simulink model "cartesianControl6Ranalytical"  (R2023b)
settings: Solver=FixedStepAuto  StartTime=0.0  StopTime=5  FixedStep=0.001  RelTol=1e-3
values from neighbouring files (symbols this model uses):
  Kp = eye(sizeTaskSpace,sizeTaskSpace)    [cartesianControl6Rmain.m]
  myRob = loadrobot("abbIrb120")    [cartesianControl6Rmain.m]
  orie_f = tform2rotm(makehgtform('yrotate',pi/2))    [cartesianControl6Rmain.m]
  orie_i = tform2rotm(initialPose)    [cartesianControl6Rmain.m]
  pe_f = [pe_f; zHeight_ideal]    [cartesianControl6Rmain.m]
  pe_i = transpose(tform2trvec(initialPose))    [cartesianControl6Rmain.m]
  q0 = configSol    [cartesianControl6Rmain.m]
  t_f = 5    [cartesianControl6Rmain.m]
  t_i = 0    [cartesianControl6Rmain.m]
undefined symbols (not defined in the file or in its folder): DiscIntNeverNeededParam
settings Model: Creator=ggi01  LastModifiedBy=ggi01
settings SolverCC: AlgebraicLoopSolver=TrustRegion
settings DebuggingCC: UnconnectedInputMsg=warning  UnconnectedOutputMsg=warning  UnconnectedLineMsg=warning
settings ModelReferenceCC: EnableRefExpFcnMdlSchedulingChecks=on
settings RTWCC: DLArmComputeVersion=19.05

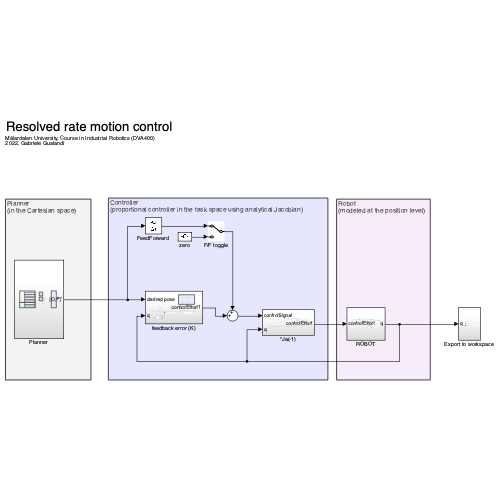
[thumbnail: Simulink's stored preview of the top-level diagram]
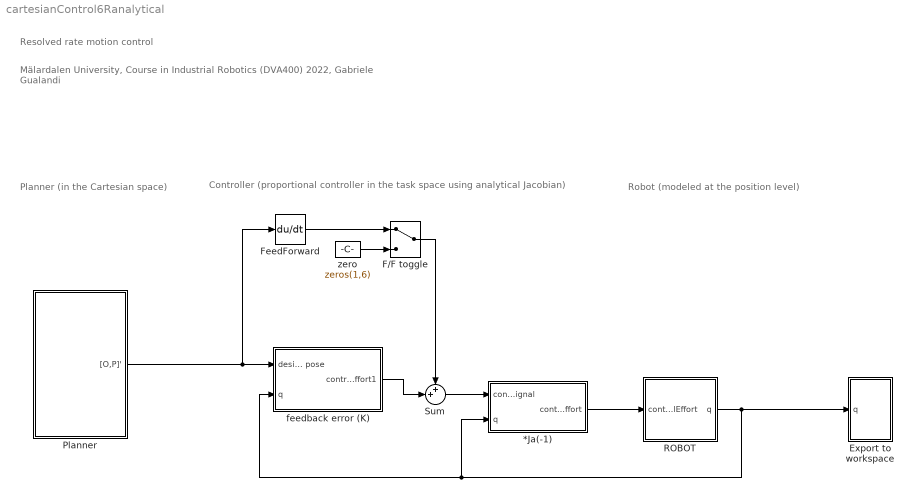
== system cartesianControl6Ranalytical ==
  note: Mälardalen University, Course in Industrial Robotics (DVA400)
      | 2022, Gabriele Gualandi
  note: Resolved rate motion control
  note: Robot
      | (modeled at the position level)
  note: Planner
      | (in the Cartesian space)
  note: Controller
      | (proportional controller in the task space using analytical Jacobian)
  *Ja(-1) : Subsystem
  Export to workspace : Subsystem
  F/F toggle : ManualSwitch
  FeedForward : Derivative
  Planner : Subsystem
  ROBOT : Subsystem
  Sum : Sum  Inputs=++|
  feedback error (K) : Subsystem
  zero : Constant  Value=zeros(1,6)
  wires:
  FeedForward/1 -> F/F toggle/1
  feedback error (K)/1(controlEffort1) -> Sum/2
  Sum/1 -> *Ja(-1)/1(controlSignal)
  *Ja(-1)/1(controlEffort) -> ROBOT/1(controlEffort)
  F/F toggle/1 -> Sum/1
  zero/1 -> F/F toggle/2
  ROBOT/1(q) -> Export to workspace/1(q), *Ja(-1)/2(q), feedback error (K)/2(q)
  Planner/1("[O,P]'") -> FeedForward/1, feedback error (K)/1(desired pose)

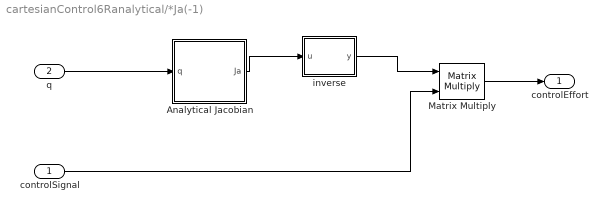
== system cartesianControl6Ranalytical/*Ja(-1) ==
  controlSignal : Inport
  q : Inport  Port=2
  Analytical Jacobian : Subsystem
  Matrix Multiply : Product  Multiplication=Matrix(*)
  inverse : MATLAB Function  TreatAsAtomicUnit=on
  controlEffort : Outport
  wires:
  q/1 -> Analytical Jacobian/1(q)
  controlSignal/1 -> Matrix Multiply/2
  inverse/1(y) -> Matrix Multiply/1
  Analytical Jacobian/1(Ja) -> inverse/1(u)
  Matrix Multiply/1 -> controlEffort/1

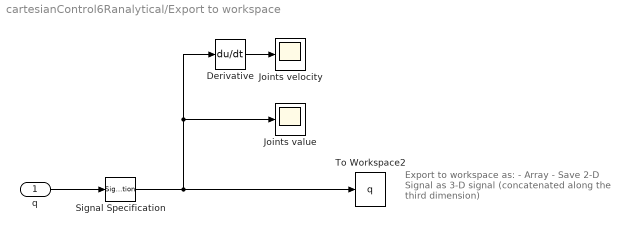
== system cartesianControl6Ranalytical/Export to workspace ==
  note: Export to workspace as:
      | - Array
      | - Save 2-D Signal as 3-D signal
      | (concatenated along the third dimension)
  q : Inport
  Derivative : Derivative
  Joints value : Scope
  Joints velocity : Scope
  Signal Specification : SignalSpecification  Dimensions=[6,1]
  To Workspace2 : ToWorkspace  VariableName=q  SampleTime=-1
  wires:
  Derivative/1 -> Joints velocity/1
  q/1 -> Signal Specification/1
  Signal Specification/1 -> Joints value/1, Derivative/1, To Workspace2/1

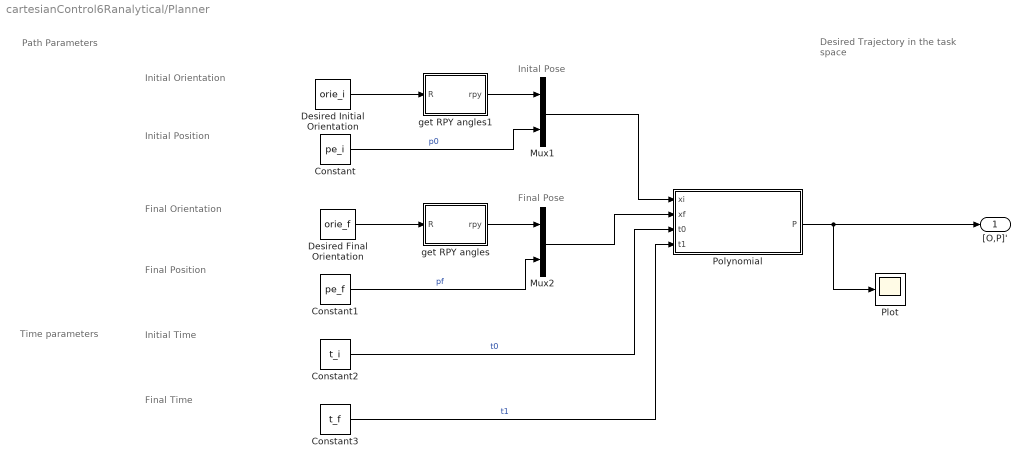
== system cartesianControl6Ranalytical/Planner ==
  note: Desired Trajectory
      | in the task space
  note: Time parameters
  note: Path Parameters
  note: Inital Pose
  note: Initial Orientation
  note: Initial Position
  note: Final Orientation
  note: Final Position
  note: Initial Time
  note: Final Time
  note: Final Pose
  Constant : Constant  Value=pe_i  VectorParams1D=off
  Constant1 : Constant  Value=pe_f  VectorParams1D=off
  Constant2 : Constant  Value=t_i
  Constant3 : Constant  Value=t_f
  Desired Final Orientation : Constant  Value=orie_f
  Desired Initial Orientation : Constant  Value=orie_i
  Mux1 : Mux  Inputs=2
  Mux2 : Mux  Inputs=2
  Plot : Scope
  Polynomial : Subsystem
  get RPY angles : MATLAB Function  TreatAsAtomicUnit=on
  get RPY angles1 : MATLAB Function  TreatAsAtomicUnit=on
  "[O,P]'" : Outport
  wires:
  Constant3/1 -> Polynomial/4(t1)  "t1"
  Constant2/1 -> Polynomial/3(t0)  "t0"
  Desired Final Orientation/1 -> get RPY angles/1(R)
  Polynomial/1(P) -> "[O,P]'"/1, Plot/1
  Desired Initial Orientation/1 -> get RPY angles1/1(R)
  Mux1/1 -> Polynomial/1(xi)
  Mux2/1 -> Polynomial/2(xf)
  get RPY angles1/1(rpy) -> Mux1/1
  Constant/1 -> Mux1/2  "p0"
  Constant1/1 -> Mux2/2  "pf"
  get RPY angles/1(rpy) -> Mux2/1

== system cartesianControl6Ranalytical/ROBOT ==
  controlEffort : Inport
  Constant : Constant  Value=q0
  Discrete-Time Integrator : DiscreteIntegrator  InitialConditionSource=external  SampleTime=-1  ICPrevOutput=DiscIntNeverNeededParam  ICPrevScaledInput=DiscIntNeverNeededParam
  Saturation : Saturate  UpperLimit=inf  LowerLimit=-inf
  q : Outport
  wires:
  Discrete-Time Integrator/1 -> q/1  "q"
  controlEffort/1 -> Saturation/1
  Constant/1 -> Discrete-Time Integrator/2
  Saturation/1 -> Discrete-Time Integrator/1

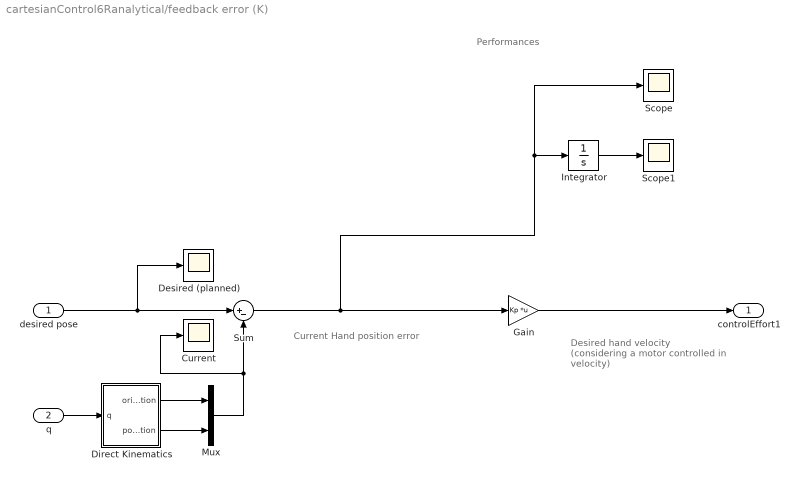
== system cartesianControl6Ranalytical/feedback error (K) ==
  note: Performances
  note: Current Hand position error
  note: Desired hand velocity
      | (considering a motor controlled
      | in velocity)
  desired pose : Inport
  q : Inport  Port=2
  Current : Scope
  Desired (planned) : Scope
  Direct Kinematics : Subsystem
  Gain : Gain  Gain=Kp  Multiplication=Matrix(K*u)
  Integrator : Integrator
  Mux : Mux  Inputs=2
  Scope : Scope
  Scope1 : Scope
  Sum : Sum  Inputs=|+-
  controlEffort1 : Outport
  wires:
  q/1 -> Direct Kinematics/1(q)
  Direct Kinematics/1(orientation) -> Mux/1
  Direct Kinematics/2(position) -> Mux/2
  desired pose/1 -> Desired (planned)/1, Sum/1
  Mux/1 -> Sum/2, Current/1
  Gain/1 -> controlEffort1/1
  Sum/1 -> Scope/1, Integrator/1, Gain/1
  Integrator/1 -> Scope1/1

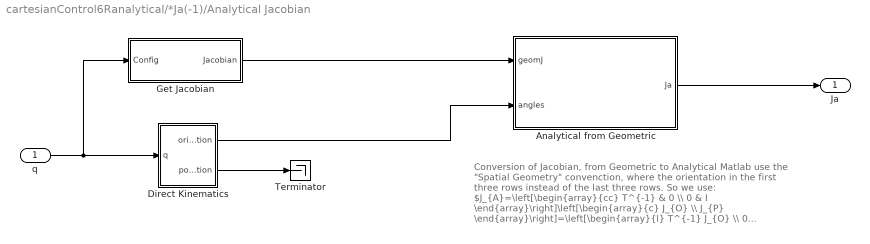
== system cartesianControl6Ranalytical/*Ja(-1)/Analytical Jacobian ==
  note: Conversion of Jacobian, from Geometric to Analytical
      |
      | Matlab use the "Spatial Geometry" convenction, where the orientation in the first three rows instead of the last three rows. So we use:
      |
      | $J_{A}=\left[\begin{array}{cc} T^{-1} & 0 \\ 0 & I \end{array}\right]\left[\begin{array}{c} J_{O} \\ J_{P} \end{array}\right]=\left[\begin{array}{l} T^{-1} J_{O} \\ 0 \end{array}\right]+\left[\begin{array}{c} 0\\ J_{P} \end{array}\right] \quad \text {if } \,\, J=\left[\begin{array}{l} J_{O} \\ J_{P} \end{array}\right]$
      |
      | If orientation is in the last three rows (as in most of the text books) we would use instead:
      |
      | $J_{A}=\left[\begin{array}{cc} I & 0 \\ 0 & T^{-1} \end{array}\right]\left[\begin{array}{c} J_{P} \\ J_{O} \end{array}\right]=\left[\begin{array}{l} J_{P} \\ 0 \end{array}\right]+\left[\begin{array}{c} 0\\ T^{-1} J_{O} \end{array}\right] \quad \text { if } \,\, J=\left[\begin{array}{l} J_{P} \\ J_{O} \end{array}\right]$
  q : Inport
  Analytical from Geometric : MATLAB Function  TreatAsAtomicUnit=on
  Direct Kinematics : Subsystem
  Get Jacobian : Subsystem  mask(Get Jacobian){RigidBodyTree=myRob, EndEffector=tool0, SimulateUsing=Code generation}
      mask prompts: RigidBodyTree "robotics:robotslmanip:blockmask:RigidBodyTreePrompt"; EndEffector "robotics:robotslmanip:blockmask:EndEffectorPrompt"; SimulateUsing "SystemBlock:MATLABSystem:SimulateUsing"
      mask help: robotics:robotslmanip:blockmask:GetJacobianDescription
      mask init:
      | try
      |    [TreeStruct, NumBodies, sysName] = robotics.slmanip.internal.block.RBTAlgorithmBlockMasks.updateMaskWorkSpaceVariables(gcb, RigidBodyTree);
      |    robotics.slmanip.internal.block.RBTAlgorithmBlockMasks.updateBlockInputDimensions(gcb, TreeStruct, 'Config');
      | catch ME
      |    TreeStruct = [];  NumBodies = [];   sysName = '???';
      |    throw(ME);
      | end
      | EndEffectorArray = robotics.slmanip.internal.block.RBTAlgorithmBlockMasks.updateBodyWSVar(gcb, RigidBodyTree, 'EndEffector');
      settings: LibrarySourceBlock=robotmaniplib/Get Jacobian
      mask Help: helpview(fullfile(docroot,'robotics','helptargets.map'), 'rstGetJacobian');
      mask TypeOptions SimulateUsing: MATLAB System/SimulateUsing
      mask DialogControl RigidBodyTree Prompt: Rigid body tree:
      mask DialogControl EndEffector Prompt: End effector:
      mask DialogControl ListControl Prompt: robotics:robotslmanip:blockmask:SelectBodyButtonPrompt
      mask DialogControl ListControl Callback: robotics.slmanip.internal.block.RBTAlgorithmBlockMasks.updateMaskBodyList(gcb, 'EndEffector');
      mask DialogControl SimulateUsing Prompt: Simulate using:
      mask DialogControl SimulateUsing Tooltip: SystemBlock:MATLABSystem:SimulateUsingDescription
      mask Display:
      | if (strcmp(sysName,'???'))
      | 	color('red');
      | else
      |     color('blue');
      | end
      | text(0.99, 0.99, sysName, 'horizontalAlignment', 'right', 'verticalAlignment','top');
      | 
      | color('black');
      | DescText = ['EE: ' get_param(gcb,'EndEffector')];
      | text(0.5, 0.05, DescText, 'horizontalAlignment', 'center', 'verticalAlignment','bottom');
      | 
      | port_label('input', 1, 'Config')
      | port_label('output', 1, 'Jacobian')
  Terminator : Terminator
  Ja : Outport
  wires:
  Direct Kinematics/1(orientation) -> Analytical from Geometric/2(angles)
  Direct Kinematics/2(position) -> Terminator/1
  Analytical from Geometric/1(Ja) -> Ja/1
  Get Jacobian/1(Jacobian) -> Analytical from Geometric/1(geomJ)
  q/1 -> Get Jacobian/1(Config), Direct Kinematics/1(q)

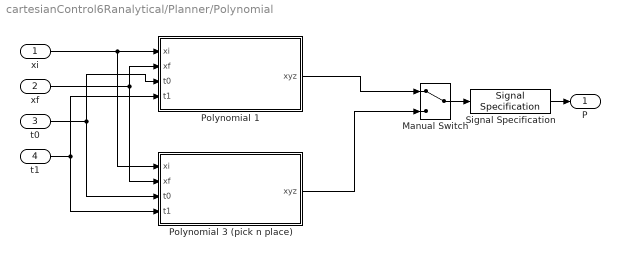
== system cartesianControl6Ranalytical/Planner/Polynomial ==
  xi : Inport
  xf : Inport  Port=2
  t0 : Inport  Port=3
  t1 : Inport  Port=4
  Manual Switch : ManualSwitch
  Polynomial 1 : Subsystem
  Polynomial 3 (pick n place) : Subsystem
  Signal Specification : SignalSpecification  OutDataTypeStr=double  Dimensions=[6,1]
  P : Outport
  wires:
  Polynomial 1/1(xyz) -> Manual Switch/1
  Polynomial 3 (pick n place)/1(xyz) -> Manual Switch/2
  xi/1 -> Polynomial 3 (pick n place)/1(xi), Polynomial 1/1(xi)
  xf/1 -> Polynomial 3 (pick n place)/2(xf), Polynomial 1/2(xf)
  t0/1 -> Polynomial 1/3(t0), Polynomial 3 (pick n place)/3(t0)
  t1/1 -> Polynomial 3 (pick n place)/4(t1), Polynomial 1/4(t1)
  Manual Switch/1 -> Signal Specification/1
  Signal Specification/1 -> P/1

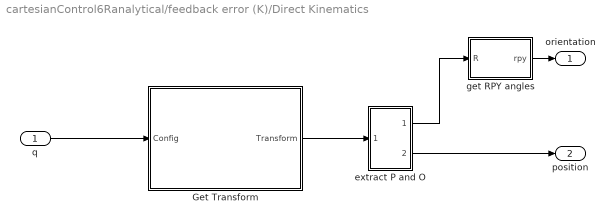
== system cartesianControl6Ranalytical/feedback error (K)/Direct Kinematics ==
  q : Inport
  Get Transform : Subsystem  mask(Get Transform){RigidBodyTree=myRob, SourceBody=tool0, TargetBody=base, SimulateUsing=Code generation}
      mask prompts: RigidBodyTree "robotics:robotslmanip:blockmask:RigidBodyTreePrompt"; SourceBody "robotics:robotslmanip:blockmask:GetTransformSourceBodyPrompt"; TargetBody "robotics:robotslmanip:blockmask:GetTransformTargetBodyPrompt"; SimulateUsing "SystemBlock:MATLABSystem:SimulateUsing"
      mask help: robotics:robotslmanip:blockmask:GetTransformDescription
      mask init:
      | try
      |    [TreeStruct, NumBodies, sysName] = robotics.slmanip.internal.block.RBTAlgorithmBlockMasks.updateMaskWorkSpaceVariables(gcb, RigidBodyTree);
      |    robotics.slmanip.internal.block.RBTAlgorithmBlockMasks.updateBlockInputDimensions(gcb, TreeStruct, 'Config');
      | catch ME
      |    TreeStruct = [];  NumBodies = [];   sysName = '???';
      |    throw(ME);
      | end
      | SourceBodyArray = robotics.slmanip.internal.block.RBTAlgorithmBlockMasks.updateBodyWSVar(gcb, RigidBodyTree, 'SourceBody');
      | TargetBodyArray = robotics.slmanip.internal.block.RBTAlgorithmBlockMasks.updateBodyWSVar(gcb, RigidBodyTree, 'TargetBody');
      settings: LibrarySourceBlock=robotmaniplib/Get Transform
      mask Help: helpview(fullfile(docroot,'robotics','helptargets.map'), 'rstGetTransform');
      mask TypeOptions SimulateUsing: MATLAB System/SimulateUsing
      mask DialogControl RigidBodyTree Prompt: Rigid body tree:
      mask DialogControl SourceBody Prompt: Source body:
      mask DialogControl ListControl1 Prompt: Select body >>
      mask DialogControl ListControl1 Callback: robotics.slmanip.internal.block.RBTAlgorithmBlockMasks.updateMaskBodyList(gcb, 'SourceBody');
      mask DialogControl TargetBody Prompt: Target body:
      mask DialogControl ListControl2 Prompt: Select body >>
      mask DialogControl ListControl2 Callback: robotics.slmanip.internal.block.RBTAlgorithmBlockMasks.updateMaskBodyList(gcb, 'TargetBody');
      mask DialogControl SimulateUsing Prompt: Simulate using:
      mask DialogControl SimulateUsing Tooltip: SystemBlock:MATLABSystem:SimulateUsingDescription
      mask Display:
      | if (strcmp(sysName,'???'))
      | 	color('red');
      | else
      |     color('blue');
      | end
      | text(0.99, 0.99, sysName, 'horizontalAlignment', 'right', 'verticalAlignment','top');
      | 
      | color('black')
      | SourceText = ['Source: ' get_param(gcb,'SourceBody')];
      | TargetText = ['Target: ' get_param(gcb,'TargetBody')];
      | DescText = [SourceText newline TargetText];
      | text(0.5, 0.05, DescText, 'horizontalAlignment', 'center','verticalAlignment','bottom');
      | 
      | port_label('input', 1, 'Config')
      | port_label('output', 1, 'Transform')
  extract P and O : Subsystem
  get RPY angles : MATLAB Function  TreatAsAtomicUnit=on
  orientation : Outport
  position : Outport  Port=2
  wires:
  get RPY angles/1(rpy) -> orientation/1
  extract P and O/1(orientation) -> get RPY angles/1(R)
  extract P and O/2(position) -> position/1
  Get Transform/1(Transform) -> extract P and O/1(In1)
  q/1 -> Get Transform/1(Config)

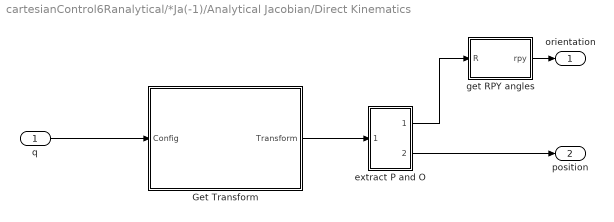
== system cartesianControl6Ranalytical/*Ja(-1)/Analytical Jacobian/Direct Kinematics ==
  q : Inport
  Get Transform : Subsystem  mask(Get Transform){RigidBodyTree=myRob, SourceBody=tool0, TargetBody=base, SimulateUsing=Code generation}
      mask prompts: RigidBodyTree "robotics:robotslmanip:blockmask:RigidBodyTreePrompt"; SourceBody "robotics:robotslmanip:blockmask:GetTransformSourceBodyPrompt"; TargetBody "robotics:robotslmanip:blockmask:GetTransformTargetBodyPrompt"; SimulateUsing "SystemBlock:MATLABSystem:SimulateUsing"
      mask help: robotics:robotslmanip:blockmask:GetTransformDescription
      mask init: same as cartesianControl6Ranalytical/feedback error (K)/Direct Kinematics/Get Transform
      settings: LibrarySourceBlock=robotmaniplib/Get Transform
      mask Help: helpview(fullfile(docroot,'robotics','helptargets.map'), 'rstGetTransform');
      mask TypeOptions SimulateUsing: MATLAB System/SimulateUsing
      mask DialogControl RigidBodyTree Prompt: Rigid body tree:
      mask DialogControl SourceBody Prompt: Source body:
      mask DialogControl ListControl1 Prompt: Select body >>
      mask DialogControl ListControl1 Callback: robotics.slmanip.internal.block.RBTAlgorithmBlockMasks.updateMaskBodyList(gcb, 'SourceBody');
      mask DialogControl TargetBody Prompt: Target body:
      mask DialogControl ListControl2 Prompt: Select body >>
      mask DialogControl ListControl2 Callback: robotics.slmanip.internal.block.RBTAlgorithmBlockMasks.updateMaskBodyList(gcb, 'TargetBody');
      mask DialogControl SimulateUsing Prompt: Simulate using:
      mask DialogControl SimulateUsing Tooltip: SystemBlock:MATLABSystem:SimulateUsingDescription
      mask Display:
      | if (strcmp(sysName,'???'))
      | 	color('red');
      | else
      |     color('blue');
      | end
      | text(0.99, 0.99, sysName, 'horizontalAlignment', 'right', 'verticalAlignment','top');
      | 
      | color('black')
      | SourceText = ['Source: ' get_param(gcb,'SourceBody')];
      | TargetText = ['Target: ' get_param(gcb,'TargetBody')];
      | DescText = [SourceText newline TargetText];
      | text(0.5, 0.05, DescText, 'horizontalAlignment', 'center','verticalAlignment','bottom');
      | 
      | port_label('input', 1, 'Config')
      | port_label('output', 1, 'Transform')
  extract P and O : Subsystem
  get RPY angles : MATLAB Function  TreatAsAtomicUnit=on
  orientation : Outport
  position : Outport  Port=2
  wires:
  get RPY angles/1(rpy) -> orientation/1
  extract P and O/1(orientation) -> get RPY angles/1(R)
  extract P and O/2(position) -> position/1
  Get Transform/1(Transform) -> extract P and O/1(In1)
  q/1 -> Get Transform/1(Config)

== system cartesianControl6Ranalytical/*Ja(-1)/Analytical Jacobian/Get Jacobian ==
  Config : Inport
  MATLAB System : MATLABSystem  System=robotics.slmanip.internal.block.GetJacobianBlock  TreeStruct=TreeStruct  EEBodyName=EndEffector  SimulateUsing=Code generation
      mask Type: robotics.slmanip.internal.block.GetJacobianBlock
      mask Display:
      | disp('GetJacobianBlock');
      | port_label('input',1,'q');
      | port_label('output',1,'jacobianMat');
  Jacobian : Outport  VectorParamsAs1DForOutWhenUnconnected=off
  wires:
  MATLAB System/1 -> Jacobian/1
  Config/1 -> MATLAB System/1

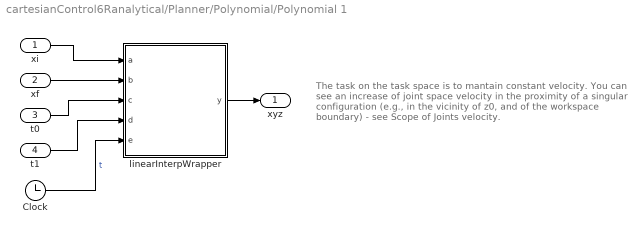
== system cartesianControl6Ranalytical/Planner/Polynomial/Polynomial 1 ==
  note: The task on the task space is to mantain constant velocity.
      | You can see an increase of joint space velocity in the proximity
      | of a singular configuration (e.g., in the vicinity of z0, and of the
      | workspace boundary) - see Scope of Joints velocity.
  xi : Inport
  xf : Inport  Port=2
  t0 : Inport  Port=3
  t1 : Inport  Port=4
  Clock : Clock
  linearInterpWrapper : MATLAB Function  TreatAsAtomicUnit=on
  xyz : Outport
  wires:
  t0/1 -> linearInterpWrapper/3(c)
  xi/1 -> linearInterpWrapper/1(a)
  xf/1 -> linearInterpWrapper/2(b)
  t1/1 -> linearInterpWrapper/4(d)
  Clock/1 -> linearInterpWrapper/5(e)  "t"
  linearInterpWrapper/1(y) -> xyz/1

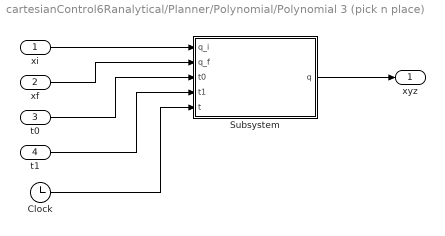
== system cartesianControl6Ranalytical/Planner/Polynomial/Polynomial 3 (pick n place) ==
  xi : Inport
  xf : Inport  Port=2
  t0 : Inport  Port=3
  t1 : Inport  Port=4
  Clock : Clock
  Subsystem : Subsystem
  xyz : Outport
  wires:
  Subsystem/1(q) -> xyz/1
  xf/1 -> Subsystem/2(q_f)
  Clock/1 -> Subsystem/5(t)
  t0/1 -> Subsystem/3(t0)
  xi/1 -> Subsystem/1(q_i)
  t1/1 -> Subsystem/4(t1)

== system cartesianControl6Ranalytical/feedback error (K)/Direct Kinematics/Get Transform ==
  Config : Inport
  MATLAB System : MATLABSystem  System=robotics.slmanip.internal.block.GetTransformBlock  TreeStruct=TreeStruct  SourceBodyName=SourceBody  TargetBodyName=TargetBody  SimulateUsing=Code generation
      mask Type: robotics.slmanip.internal.block.GetTransformBlock
      mask Display:
      | disp('GetTransformBlock');
      | port_label('input',1,'q');
      | port_label('output',1,'tform');
  Transform : Outport  VectorParamsAs1DForOutWhenUnconnected=off
  wires:
  MATLAB System/1 -> Transform/1
  Config/1 -> MATLAB System/1

== system cartesianControl6Ranalytical/feedback error (K)/Direct Kinematics/extract P and O ==
  In1 : Inport
  Orientation : MATLABFcn  MATLABFcn=tform2rotm  Output1D=off
  Position : MATLABFcn  MATLABFcn=tform2trvec
  orientation : Outport
  position : Outport  Port=2
  wires:
  Orientation/1 -> orientation/1
  In1/1 -> Position/1, Orientation/1
  Position/1 -> position/1

== system cartesianControl6Ranalytical/*Ja(-1)/Analytical Jacobian/Direct Kinematics/Get Transform ==
  Config : Inport
  MATLAB System : MATLABSystem  System=robotics.slmanip.internal.block.GetTransformBlock  TreeStruct=TreeStruct  SourceBodyName=SourceBody  TargetBodyName=TargetBody  SimulateUsing=Code generation
      mask Type: robotics.slmanip.internal.block.GetTransformBlock
      mask Display:
      | disp('GetTransformBlock');
      | port_label('input',1,'q');
      | port_label('output',1,'tform');
  Transform : Outport  VectorParamsAs1DForOutWhenUnconnected=off
  wires:
  MATLAB System/1 -> Transform/1
  Config/1 -> MATLAB System/1

== system cartesianControl6Ranalytical/*Ja(-1)/Analytical Jacobian/Direct Kinematics/extract P and O ==
  In1 : Inport
  Orientation : MATLABFcn  MATLABFcn=tform2rotm  Output1D=off
  Position : MATLABFcn  MATLABFcn=tform2trvec
  orientation : Outport
  position : Outport  Port=2
  wires:
  Orientation/1 -> orientation/1
  In1/1 -> Position/1, Orientation/1
  Position/1 -> position/1

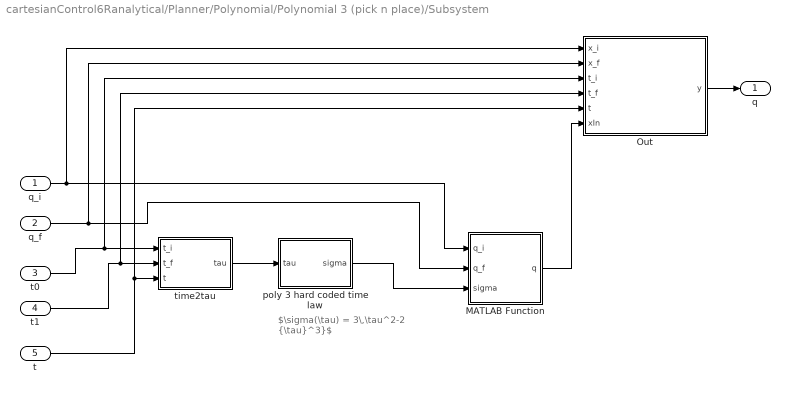
== system cartesianControl6Ranalytical/Planner/Polynomial/Polynomial 3 (pick n place)/Subsystem ==
  note: $\sigma(\tau) = 3\,\tau^2-2 {\tau}^3}$
  q_i : Inport
  q_f : Inport  Port=2
  t0 : Inport  Port=3
  t1 : Inport  Port=4
  t : Inport  Port=5
  MATLAB Function : MATLAB Function  TreatAsAtomicUnit=on
  Out : MATLAB Function  TreatAsAtomicUnit=on
  poly 3 hard coded time law : MATLAB Function  TreatAsAtomicUnit=on
  time2tau : MATLAB Function  TreatAsAtomicUnit=on
  q : Outport
  wires:
  q_f/1 -> Out/2(x_f), MATLAB Function/2(q_f)
  t/1 -> Out/5(t), time2tau/3(t)
  t0/1 -> Out/3(t_i), time2tau/1(t_i)
  MATLAB Function/1(q) -> Out/6(xIn)
  t1/1 -> Out/4(t_f), time2tau/2(t_f)
  q_i/1 -> Out/1(x_i), MATLAB Function/1(q_i)
  time2tau/1(tau) -> poly 3 hard coded time law/1(tau)
  poly 3 hard coded time law/1(sigma) -> MATLAB Function/3(sigma)
  Out/1(y) -> q/1

== matlab function cartesianControl6Ranalytical/Planner/Polynomial/Polynomial 3 (pick n place)/Subsystem/Out ==
  data: x_i input; y output; x_f input; t_i input; t_f input; t input; xIn input
function y = intervalGuardWrapper(x_i, x_f, t_i, t_f, t, xIn )

y = intervalGuard(x_i, x_f, t_i, t_f, t, xIn );

== matlab function cartesianControl6Ranalytical/*Ja(-1)/inverse ==
  data: u input; y output
function y = fcn(u)

y = inv(u);

== matlab function cartesianControl6Ranalytical/*Ja(-1)/Analytical Jacobian/Direct Kinematics/get RPY angles ==
  data: R input; rpy output
function rpy = rpyWrap(R)
%rpy = getRPYanglesFromR(R);
[rpy, ~] = eulerInverseProblem(R,'zyx','current');

== matlab function cartesianControl6Ranalytical/Planner/get RPY angles1 ==
  data: R input; rpy output
function rpy = rpyWrap(R)

%rpy = getRPYanglesFromR(R);
[rpy, ~] = eulerInverseProblem(R);

== matlab function cartesianControl6Ranalytical/*Ja(-1)/Analytical Jacobian/Analytical from Geometric ==
  data: geomJ input; Ja output; angles input
function Ja = JacobAnFromGeomWrapper(geomJ,angles)
% For T^-1 matrix using RPY i.e., z(r) y(p) x(y) wrt to the current frame

T = rpy2Tmatrix(angles);

Tinv = inv(T);

% Following matlab convention (Jo is on top of Jp)
Ja = [Tinv,zeros(3);zeros(3),eye(3)] * geomJ;

% In standard convention one would have:
% analytJ = [eye(3),zeros(3);zeros(3),Tinv] * geomJ;

== matlab function cartesianControl6Ranalytical/feedback error (K)/Direct Kinematics/get RPY angles ==
  data: R input; rpy output
function rpy = rpyWrap(R)
%rpy = getRPYanglesFromR(R);
[rpy, ~] = eulerInverseProblem(R,'zyx','current');

== matlab function cartesianControl6Ranalytical/Planner/Polynomial/Polynomial 3 (pick n place)/Subsystem/MATLAB Function ==
  data: q_i input; q output; q_f input; sigma input
function q = fcn(q_i,q_f,sigma)

h = q_f - q_i;
q = q_i + h * sigma;

== matlab function cartesianControl6Ranalytical/Planner/get RPY angles ==
  data: R input; rpy output
function rpy = rpyWrap(R)

[rpy, ~] = eulerInverseProblem( R );

== matlab function cartesianControl6Ranalytical/Planner/Polynomial/Polynomial 1/linearInterpWrapper ==
  data: a input; y output; b input; c input; d input; e input
function y = linearInterpWrapper(a,b,c,d,e)

y = linearInterp(a,b,c,d,e);

== matlab function cartesianControl6Ranalytical/Planner/Polynomial/Polynomial 3 (pick n place)/Subsystem/poly 3 hard coded time law ==
  data: tau input; sigma output
function sigma = fcn(tau)

sigma = 3 * tau^2 - 2 * tau^3;

== matlab function cartesianControl6Ranalytical/Planner/Polynomial/Polynomial 3 (pick n place)/Subsystem/time2tau ==
  data: t_i input; t_f input; t input; tau output
function tau = t2tau(t_i,t_f,t)
T = t_f - t_i;
tau = (t - t_i)/T;
